simulink model "TriggerFun2_2018a"  (R2018a)
settings: Solver=VariableStepAuto  StartTime=0.0  StopTime=0.5  FixedStep=1  MaxStep=1  RelTol=1e-3
settings Model: Creator=86188  LastModifiedBy=bzhan

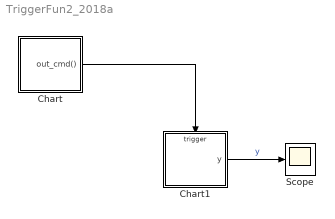
== system TriggerFun2_2018a ==
  Chart : Stateflow chart  TreatAsAtomicUnit=on
  Chart1 : Stateflow chart  TreatAsAtomicUnit=on
  Scope : Scope
  wires:
  Chart/1(out_cmd()) -> Chart1/Trigger
  Chart1/1(y) -> Scope/1  "y"

== stateflow chart TriggerFun2_2018a/Chart1 ==
  settings: executeAtInitialization=1
  state AA
    du: y = y + 1;
  (default) -> AA
  data: y output =0
  events: out_cmd input FUNCTION_CALL_EVENT

== stateflow chart TriggerFun2_2018a/Chart ==
  settings: updateMethod=DISCRETE  sampleTime=0.1
  state ENTRY
    en:f("en_ENTRY");
  state A
    en:
    f("en_A");
    send(out_cmd);
    send(out_cmd);
    send(out_cmd);
    send(out_cmd);
  state B
  (default) -> ENTRY
  A -> B
  ENTRY -> A
  data: s function_input
  events: out_cmd output FUNCTION_CALL_EVENT
  function f(s):
    | function f(s)
    |   fprintf(s+"\n");
